simulink model "proyecto_simulink"  (R2023a)
settings: Solver=VariableStepAuto  StartTime=0.0  StopTime=20  RelTol=1e-3
settings Model: Creator=nicol  LastModifiedBy=nicol

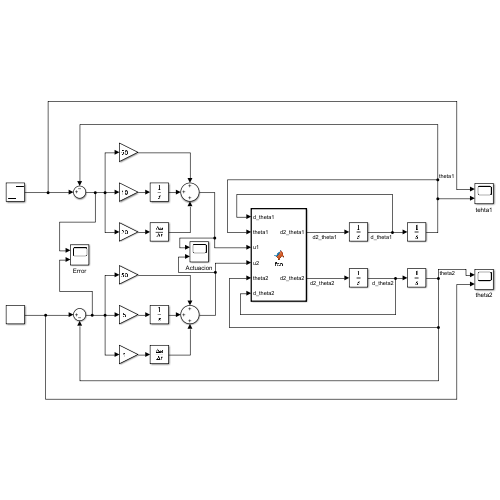
[thumbnail: Simulink's stored preview of the top-level diagram]
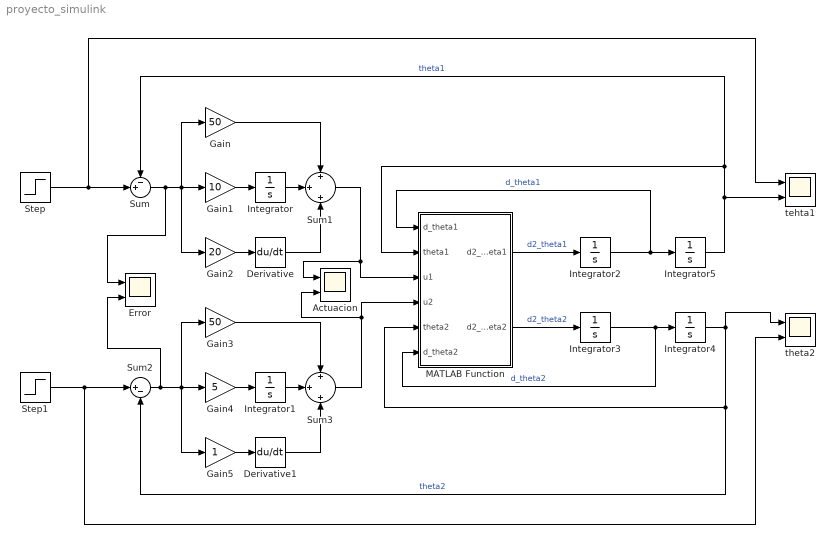
== system proyecto_simulink ==
  Actuacion : Scope  NumInputPorts=2
  Derivative : Derivative
  Derivative1 : Derivative
  Error : Scope  NumInputPorts=2
  Gain : Gain  Gain=50
  Gain1 : Gain  Gain=10
  Gain2 : Gain  Gain=20
  Gain3 : Gain  Gain=50
  Gain4 : Gain  Gain=5
  Gain5 : Gain
  Integrator{,1..5} (6 alike) : Integrator
  MATLAB Function : MATLAB Function  TreatAsAtomicUnit=on
  Step : Step  Time=0  After=pi/2  SampleTime=0
  Step1 : Step  Time=0  After=0  SampleTime=0
  Sum : Sum  Inputs=-+|
  Sum1 : Sum  Inputs=+|+|+
  Sum2 : Sum  Inputs=|+-
  Sum3 : Sum  Inputs=+|+|+
  tehta1 : Scope  NumInputPorts=2
  theta2 : Scope  NumInputPorts=2
  wires:
  Gain2/1 -> Derivative/1
  Gain1/1 -> Integrator/1
  Integrator/1 -> Sum1/2
  Gain/1 -> Sum1/1
  Derivative/1 -> Sum1/3
  Sum/1 -> Error/1, Gain2/1, Gain1/1, Gain/1
  MATLAB Function/1(d2_theta1) -> Integrator2/1  "d2_theta1"
  Step1/1 -> theta2/2, Sum2/1
  MATLAB Function/2(d2_theta2) -> Integrator3/1  "d2_theta2"
  Integrator2/1 -> MATLAB Function/1(d_theta1), Integrator5/1  "d_theta1"
  Integrator3/1 -> MATLAB Function/6(d_theta2), Integrator4/1  "d_theta2"
  Integrator4/1 -> theta2/1, Sum2/2, MATLAB Function/5(theta2)  "theta2"
  Integrator5/1 -> tehta1/2, Sum/1, MATLAB Function/2(theta1)  "theta1"
  Gain4/1 -> Integrator1/1
  Integrator1/1 -> Sum3/2
  Gain5/1 -> Derivative1/1
  Derivative1/1 -> Sum3/3
  Gain3/1 -> Sum3/1
  Sum2/1 -> Error/2, Gain5/1, Gain3/1, Gain4/1
  Sum3/1 -> MATLAB Function/4(u2), Actuacion/2
  Sum1/1 -> MATLAB Function/3(u1), Actuacion/1
  Step/1 -> tehta1/1, Sum/2

== matlab function proyecto_simulink/MATLAB Function ==
  data: d_theta1 input; theta1 input; u1 input; u2 input; theta2 input; d_theta2 input; d2_theta1 output; d2_theta2 output
function [d2_theta1, d2_theta2] = fcn(d_theta1, theta1, u1, u2, theta2, d_theta2)

    M1 = 1;
    M2 = 1;
    L1 = 1;
    L2 = 1;
    g = 9.8;

    B = [(M1 + M2)*L2^2 + M2*L2^2 + 2*M2*L1*L2*cos(theta2), M2*L2^2 + M2*L1*L2*cos(theta2);
         M2*L2^2 + M2*L1*L2*cos(theta2),                   M2*L2^2];


    Cm = [-M2*L1*L2*sin(theta2)*(2*d_theta1*d_theta2 + d_theta2^2);
          M2*L1*L2*sin(theta2)*d_theta1^2];

    G = [(M1 + M2)*g*L1*cos(theta1) + M2*g*L2*cos(theta1 + theta2);
         M2*g*L2*cos(theta1 + theta2)];

    F = [u1; u2];

    aux = F - Cm - G;

    result = B\aux;

    d2_theta1 = result(1);
    d2_theta2 = result(2);
end
